simulink model "so3_ballpark"  (R2024b)
settings: Solver=FixedStepAuto  StartTime=0.0  StopTime=80  FixedStep=0.0001  RelTol=1e-3
values from neighbouring files (symbols this model uses):
  cube_length = 0.3    [s03_ballpark_init.m]
  cube_mass = 3    [s03_ballpark_init.m]
  Kr = 0.3    [s03_ballpark_init.m]
  Kw = 0.5*Kr    (= 0.15)    [s03_ballpark_init.m]
  q_des = eul2quat(desiered_rot_euler)    [s03_ballpark_init.m]
  T = 0.05    [s03_ballpark_init.m]    (also in thruster_mapper.m = 0.1)
  thruster_matrix = [ ... (first row only)    [s03_ballpark_init.m]    (also in thruster_mapper.m)
  X_0 = [ ... (first row only)    [s03_ballpark_init.m]
undefined symbols (not defined in the file or in its folder): X, Y, Z
libraries: simulink x24, nesl_utility x18, sm_lib x5
settings Model: Creator=user  LastModifiedBy=user
settings OptimizationCC: BlockReduction=off  DefaultParameterBehavior=Inlined  BufferReuse=off

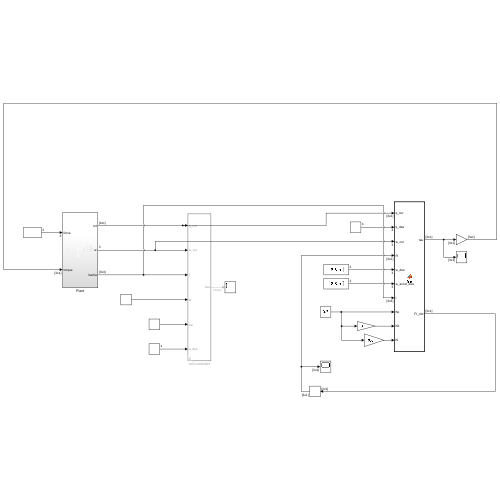
[thumbnail: Simulink's stored preview of the top-level diagram]
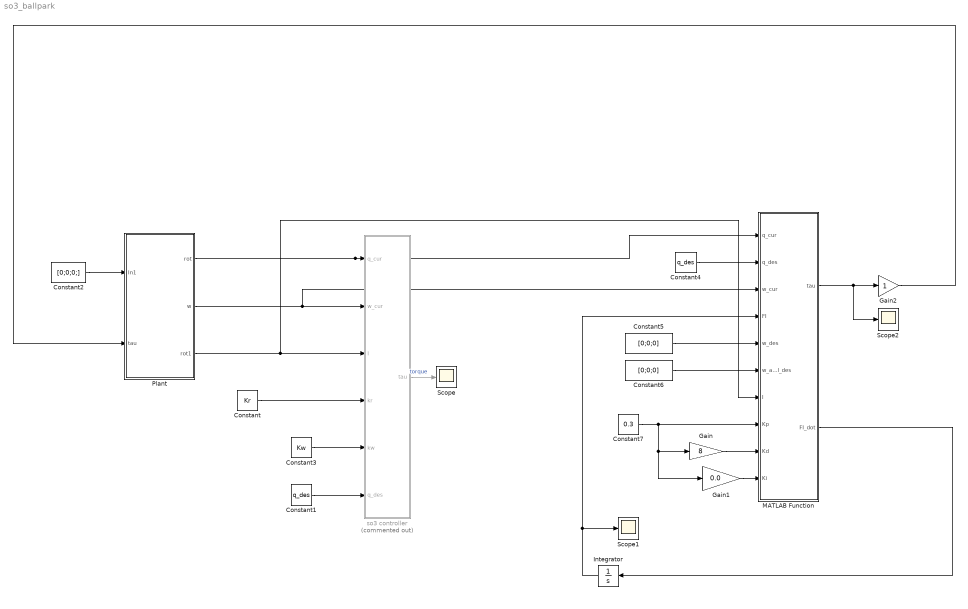
== system so3_ballpark ==
  Constant : Constant  Value=Kr
  Constant1 : Constant  Value=q_des
  Constant2 : Constant  Value=[0;0;0;]
  Constant3 : Constant  Value=Kw
  Constant4 : Constant  Value=q_des
  Constant5 : Constant  Value=[0;0;0]
  Constant6 : Constant  Value=[0;0;0]
  Constant7 : Constant  Value=0.3
  Gain : Gain  Gain=8
  Gain1 : Gain  Gain=0.0
  Gain2 : Gain
  Integrator : Integrator  InitialCondition=[0;0;0]
  MATLAB Function : MATLAB Function  TreatAsAtomicUnit=on  SystemSampleTime=T
  Plant : Subsystem
  Scope : Scope
  Scope1 : Scope
  Scope2 : Scope
  so3 controller : MATLAB Function  Commented=on  TreatAsAtomicUnit=on
  wires:
  so3 controller/1(tau) -> Scope/1  "torque"
  Plant/1(rot) -> MATLAB Function/1(q_cur), so3 controller/1(q_cur)
  Plant/2(w) -> MATLAB Function/3(w_cur), so3 controller/2(w_cur)
  Constant/1 -> so3 controller/4(kr)
  Constant1/1 -> so3 controller/6(q_des)
  Plant/3(rot1) -> MATLAB Function/7(I), so3 controller/3(I)
  Constant2/1 -> Plant/1(In1)
  Constant3/1 -> so3 controller/5(kw)
  MATLAB Function/2(FI_dot) -> Integrator/1
  Integrator/1 -> Scope1/1, MATLAB Function/4(FI)
  Constant4/1 -> MATLAB Function/2(q_des)
  Constant5/1 -> MATLAB Function/5(w_des)
  Constant6/1 -> MATLAB Function/6(w_accel_des)
  Constant7/1 -> Gain1/1, Gain/1, MATLAB Function/8(Kp)
  Gain/1 -> MATLAB Function/9(Kd)
  Gain1/1 -> MATLAB Function/10(Ki)
  MATLAB Function/1(tau) -> Scope2/1, Gain2/1
  Gain2/1 -> Plant/2(tau)

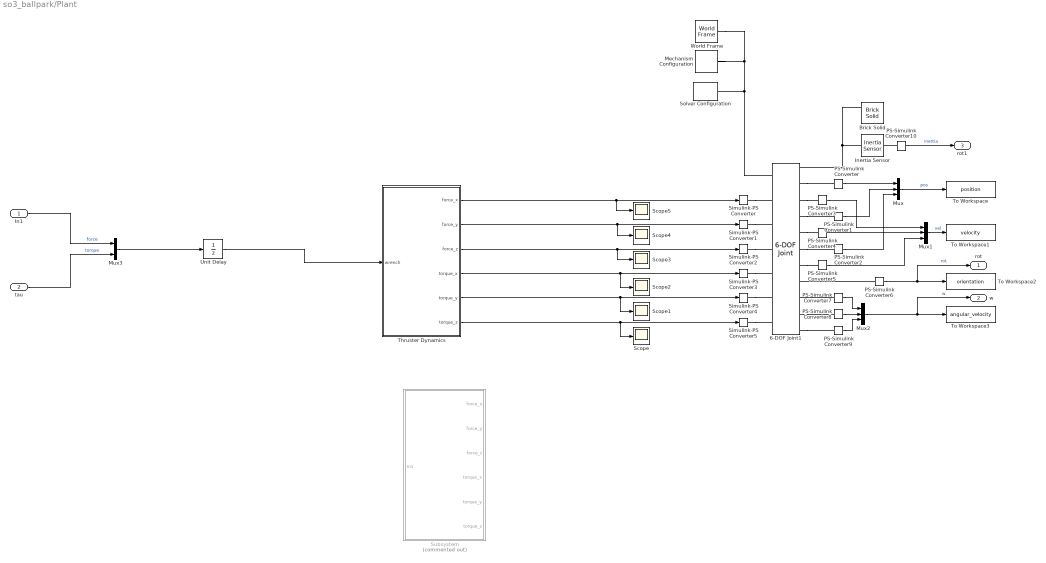
== system so3_ballpark/Plant ==
  In1 : Inport
  tau : Inport  Port=2
  6-DOF Joint1 : sm_lib/Joints/6-DOF Joint  JointMode=Normal  CompositeWrenchDir=FollowerOnBase  CompositeWrenchFrame=BaseFrame  SenseConstraintForce=off  SenseConstraintTorque=off  SenseTotalForce=off  SenseTotalTorque=off  PxPositionTargetSpecify=on  PxPositionTargetPriority=High  PxPositionTargetValue=X_0(1)  PxPositionTargetValueUnits=m  PxVelocityTargetSpecify=on  PxVelocityTargetPriority=High  PxVelocityTargetValue=X_0(4)  PxVelocityTargetValueUnits=m/s  PxEquilibriumPosition=0  PxEquilibriumPositionUnits=m  PxSpringStiffness=0  PxSpringStiffnessUnits=N/m  PxDampingCoefficient=0  PxDampingCoefficientUnits=N/(m/s)  PxLowerLimitSpecify=off  PxLowerLimitBound=-1  PxLowerLimitBoundUnits=m  PxLowerLimitStiffness=1e6  PxLowerLimitStiffnessUnits=N/m  PxLowerLimitDamping=1e3  PxLowerLimitDampingUnits=N/(m/s)  PxLowerLimitTransitionRegionWidth=1e-4  PxLowerLimitTransitionRegionWidthUnits=m  PxUpperLimitSpecify=off  PxUpperLimitBound=1  PxUpperLimitBoundUnits=m  PxUpperLimitStiffness=1e6  PxUpperLimitStiffnessUnits=N/m  PxUpperLimitDamping=1e3  PxUpperLimitDampingUnits=N/(m/s)  PxUpperLimitTransitionRegionWidth=1e-4  PxUpperLimitTransitionRegionWidthUnits=m  PxTorqueActuationMode=InputTorque  PxMotionActuationMode=ComputedMotion  PxSensePosition=on  PxSenseVelocity=on  PxSenseAcceleration=off  PxSenseTorqueForce=off  PxSenseLowerLimitTorqueForce=off  PxSenseUpperLimitTorqueForce=off  PyPositionTargetSpecify=on  PyPositionTargetPriority=High  PyPositionTargetValue=X_0(2)  PyPositionTargetValueUnits=m  PyVelocityTargetSpecify=on  PyVelocityTargetPriority=High  PyVelocityTargetValue=X_0(5)  PyVelocityTargetValueUnits=m/s  PyEquilibriumPosition=0  PyEquilibriumPositionUnits=m  PySpringStiffness=0  PySpringStiffnessUnits=N/m  PyDampingCoefficient=0  PyDampingCoefficientUnits=N/(m/s)  PyLowerLimitSpecify=off  PyLowerLimitBound=-1  PyLowerLimitBoundUnits=m  PyLowerLimitStiffness=1e6  PyLowerLimitStiffnessUnits=N/m  PyLowerLimitDamping=1e3  PyLowerLimitDampingUnits=N/(m/s)  PyLowerLimitTransitionRegionWidth=1e-4  PyLowerLimitTransitionRegionWidthUnits=m  PyUpperLimitSpecify=off  PyUpperLimitBound=1  PyUpperLimitBoundUnits=m  PyUpperLimitStiffness=1e6  PyUpperLimitStiffnessUnits=N/m  PyUpperLimitDamping=1e3  PyUpperLimitDampingUnits=N/(m/s)  PyUpperLimitTransitionRegionWidth=1e-4  PyUpperLimitTransitionRegionWidthUnits=m  PyTorqueActuationMode=InputTorque  PyMotionActuationMode=ComputedMotion  PySensePosition=on  PySenseVelocity=on  PySenseAcceleration=off  PySenseTorqueForce=off  PySenseLowerLimitTorqueForce=off  PySenseUpperLimitTorqueForce=off  PzPositionTargetSpecify=on  PzPositionTargetPriority=High  PzPositionTargetValue=X_0(3)  PzPositionTargetValueUnits=m  PzVelocityTargetSpecify=on  PzVelocityTargetPriority=High  PzVelocityTargetValue=X_0(6)  PzVelocityTargetValueUnits=m/s  PzEquilibriumPosition=0  PzEquilibriumPositionUnits=m  PzSpringStiffness=0  PzSpringStiffnessUnits=N/m  PzDampingCoefficient=0  PzDampingCoefficientUnits=N/(m/s)  PzLowerLimitSpecify=off  PzLowerLimitBound=-1  PzLowerLimitBoundUnits=m  PzLowerLimitStiffness=1e6  PzLowerLimitStiffnessUnits=N/m  PzLowerLimitDamping=1e3  PzLowerLimitDampingUnits=N/(m/s)  PzLowerLimitTransitionRegionWidth=1e-4  PzLowerLimitTransitionRegionWidthUnits=m  PzUpperLimitSpecify=off  PzUpperLimitBound=1  PzUpperLimitBoundUnits=m  PzUpperLimitStiffness=1e6  PzUpperLimitStiffnessUnits=N/m  PzUpperLimitDamping=1e3  PzUpperLimitDampingUnits=N/(m/s)  PzUpperLimitTransitionRegionWidth=1e-4  PzUpperLimitTransitionRegionWidthUnits=m  PzTorqueActuationMode=InputTorque  PzMotionActuationMode=ComputedMotion  PzSensePosition=on  PzSenseVelocity=on  PzSenseAcceleration=off  PzSenseTorqueForce=off  PzSenseLowerLimitTorqueForce=off  PzSenseUpperLimitTorqueForce=off  SphPositionTargetSpecify=on  SphPositionTargetPriority=High  SphPositionTargetRotationMethod=RotationSequence  SphPositionTargetFollAlignAxisA=+X  SphPositionTargetBaseAlignAxisA=+Y  SphPositionTargetFollAlignAxisB=+Y  SphPositionTargetBaseAlignAxisB=+Z  SphPositionTargetRotationStandardAxis=+Z  SphPositionTargetRotationAngle=0  SphPositionTargetRotationAngleUnits=deg  SphPositionTargetRotationArbitraryAxis=[0 0 1]  SphPositionTargetRotationSequenceAxes=FollowerAxes  SphPositionTargetRotationSequence=XYZ  SphPositionTargetRotationSequenceAngles=X_0(7:9)'  SphPositionTargetRotationSequenceAnglesUnits=deg  SphPositionTargetRotationMatrix=[1 0 0;0 1 0;0 0 1]  SphPositionTargetQuaternion=[1 0 0 0]  SphVelocityTargetSpecify=on  SphVelocityTargetPriority=High  SphVelocityTargetValue=X_0(10:12)'  SphVelocityTargetValueUnits=deg/s  SphVelocityTargetInFollowerFrame=on  SphEqPosRotationMethod=None  SphEqPosFollAlignAxisA=+X  SphEqPosBaseAlignAxisA=+Y  SphEqPosFollAlignAxisB=+Y  SphEqPosBaseAlignAxisB=+Z  SphEqPosRotationStandardAxis=+Z  SphEqPosRotationAngle=0  SphEqPosRotationAngleUnits=deg  SphEqPosRotationArbitraryAxis=[0 0 1]  SphEqPosRotationSequenceAxes=FollowerAxes  SphEqPosRotationSequence=XYX  SphEqPosRotationSequenceAngles=[0 0 0]  SphEqPosRotationSequenceAnglesUnits=deg  SphEqPosRotationMatrix=[1 0 0;0 1 0;0 0 1]  SphEqPosQuaternion=[1 0 0 0]  SphSpringStiffness=0  SphSpringStiffnessUnits=N*m/deg  SphDampingCoefficient=0  SphDampingCoefficientUnits=N*m/(deg/s)  SphLowerLimitSpecify=off  SphLowerLimitBound=15  SphLowerLimitBoundUnits=deg  SphLowerLimitStiffness=1e4  SphLowerLimitStiffnessUnits=N*m/deg  SphLowerLimitDamping=10  SphLowerLimitDampingUnits=N*m/(deg/s)  SphLowerLimitTransitionRegionWidth=0.1  SphLowerLimitTransitionRegionWidthUnits=deg  SphUpperLimitSpecify=off  SphUpperLimitBound=45  SphUpperLimitBoundUnits=deg  SphUpperLimitStiffness=1e4  SphUpperLimitStiffnessUnits=N*m/deg  SphUpperLimitDamping=10  SphUpperLimitDampingUnits=N*m/(deg/s)  SphUpperLimitTransitionRegionWidth=0.1  SphUpperLimitTransitionRegionWidthUnits=deg  SphTorqueActuationMode=InputTorque  SphActuateTorqueX=on  SphActuateTorqueY=on  SphActuateTorqueZ=on  SphActuateTorque=off  SphActuationFrame=BaseFrame  SphSensePosition=on  SphSenseVelocityX=on  SphSenseVelocityY=on  SphSenseVelocityZ=on  SphSenseVelocity=off  SphSenseAccelerationX=off  SphSenseAccelerationY=off  SphSenseAccelerationZ=off  SphSenseAcceleration=off  SphSenseLowerLimitTorqueMag=off  SphSenseUpperLimitTorqueMag=off  SphSensingFrame=BaseFrame
  Brick Solid : sm_lib/Body Elements/Brick Solid  BrickDimensions=[cube_length cube_length cube_length]  BrickDimensionsUnits=m  ExportEntireGeometry=on  InertiaType=CalculateFromGeometry  BasedOnType=Mass  Density=1000  DensityUnits=kg/m^3  Mass=cube_mass  MassUnits=kg  CenterOfMass=[0 0 0]  CenterOfMassUnits=m  MomentsOfInertia=[1 1 1]  MomentsOfInertiaUnits=kg*m^2  ProductsOfInertia=[0 0 0]  ProductsOfInertiaUnits=kg*m^2  GraphicType=FromGeometry  MarkerShape=Sphere  MarkerSize=10  GraphicVisPropType=SimpleVisualProperties  GraphicDiffuseColor=[0.5 0.5 0.5]  GraphicOpacity=1  GraphicSpecularColor=[0.5 0.5 0.5 1.0]  GraphicAmbientColor=[0.15 0.15 0.15 1.0]  GraphicEmissiveColor=[0.0 0.0 0.0 1.0]  GraphicShininess=75  DoExposeReferenceFrame=on  SerializedFrames=<Frames><Frame><Id>Frame1</Id><Value><Name>F1</Name><Origin><Source>ReferenceFrame</Source><FeatureName></FeatureName></Origin><PrimaryAxis><DefinedDirection>+Z</DefinedDirection><Source>ReferenceFrame</Source><SourceDirection>+Z</SourceDirection><FeatureName></FeatureName></PrimaryAxis><SecondaryAxis><DefinedDirection>+X</DefinedDirection><Source>ReferenceFrame</Source><SourceDirection>+X</SourceDirection><FeatureName></FeatureName></SecondaryAxis></Value></Frame></Frames>
  Inertia Sensor : sm_lib/Body Elements/Inertia Sensor  SensorExtent=BodyGroup  SpanWeldJoints=off  ExcludeGroundedBodies=off  MeasurementFrame=Attached  SenseMass=off  SenseCenterOfMass=off  SenseInertiaMatrix=on  SenseCenteredInertiaMatrix=off  SensePrincipalInertiaMatrix=off  SenseRotationMatrix=off  GraphicType=PrincipalInertiaFrame  PrincipalInertiaFrameSize=20  GraphicVisPropType=SimpleVisualProperties  GraphicDiffuseColor=[0.5 0.5 0.5]  GraphicOpacity=1  GraphicSpecularColor=[0.5 0.5 0.5 1.0]  GraphicAmbientColor=[0.15 0.15 0.15 1.0]  GraphicEmissiveColor=[0.0 0.0 0.0 1.0]  GraphicShininess=75
  Mechanism Configuration : sm_lib/Utilities/Mechanism Configuration  UniformGravity=Constant  GravityVector=[0 0 0]  GravityVectorUnits=m/s^2  LinearizationDelta=0.001  JointModeTransitionNonlinearIterations=2
  Mux : Mux  Inputs=3
  Mux1 : Mux  Inputs=3
  Mux2 : Mux  Inputs=3
  Mux3 : Mux  Inputs=2
  PS-Simulink Converter{,1..10} (11 alike) : nesl_utility/PS-Simulink Converter  PhysicalDomain=network_engine_domain  SubClassName=ps_output  LeftPortType=input  RightPortType=output  PseudoPeriodic=off  Frequencies=[]  VectorFormat=inherit  Unit=inherit  AffineConversion=off
  Scope{,1..5} (6 alike) : Scope
  Simulink-PS Converter{,1..5} (6 alike) : nesl_utility/Simulink-PS Converter  PhysicalDomain=network_engine_domain  SubClassName=ps_input  LeftPortType=input  RightPortType=output  PseudoPeriodic=off  Frequencies=[]  NoiseDistribution=none  NoiseParameters=[]  Unit=1  AffineConversion=off  FilteringAndDerivatives=provide  SimscapeFilterOrder=1  InputFilterTimeConstant=0.001  UdotUserProvided=0
  Solver Configuration : nesl_utility/Solver Configuration  PhysicalDomain=network_engine_domain  SubClassName=solver  LeftPortType=input  RightPortType=generic  Tones=[]  Harmonics=[]  SimulateNoise=off  Profile=off  UseLocalSampling=off  EnableSwitchedLinearOptims=on  FrequencyDomain=off  UseCCode=off  RelTol=0.001  AbsTol=0.001  MinStep=1e-09  ToWorkspace=off  RevertToSquareIcSolve=off  NumHomotopyIterations=100  PhasorMode=off  PhasorModeNumHarmonics=1  ConsistencySolver=NEWTON_XTOL_AFTER_FTOL  IndexReductionMethod=DerivativeReplacement  DoDC=off  ResidualTolerance=1e-09  ConsistencyTolSource=GLOBAL  ConsistencyAbsTol=0.001  ConsistencyRelTol=0.001  ConsistencyTolFactor=0.001  UseLocalSolver=off  LocalSolverChoice=NE_BACKWARD_EULER_ADVANCER  ResolveIndetEquations=on  FunctionEvalNumThread=1  LocalSolverSampleTime=0.001  DoFixedCost=off  MaxNonlinIter=3  MaxModeIter=2  ComputeImpulses=off  ImpulseIterations=2  LinearAlgebra=auto  LinearAlgebraNumThread=0  EquationFormulation=NE_TIME_EF  DelaysMemoryBudget=1024  AutomaticFiltering=on  FilteringTimeConstant=0.001  PartitionStorageMethod=AS_NEEDED  PartitionMemoryBudget=1024  PartitionMethod=ROBUST  MultibodyUseLocalSolver=off  MultibodyLocalSolverChoice=ODE1  MultibodyLocalSolverSampleTime=0.001
  Subsystem : Subsystem  Commented=on
  Thruster Dynamics : Subsystem
  To Workspace : ToWorkspace  VariableName=position  SampleTime=-1
  To Workspace1 : ToWorkspace  VariableName=velocity  SampleTime=-1
  To Workspace2 : ToWorkspace  VariableName=orientation  SampleTime=-1
  To Workspace3 : ToWorkspace  VariableName=angular_velocity  SampleTime=-1
  Unit Delay : UnitDelay  SampleTime=-1  HasFrameUpgradeWarning=on
  World Frame : sm_lib/Frames and Transforms/World Frame
  rot : Outport
  w : Outport  Port=2
  rot1 : Outport  Port=3
  wires:
  PS-Simulink Converter4/1 -> Mux1/2
  Mux1/1 -> To Workspace1/1  "vel"
  PS-Simulink Converter5/1 -> Mux1/3
  PS-Simulink Converter8/1 -> Mux2/2
  Mux/1 -> To Workspace/1  "pos"
  PS-Simulink Converter9/1 -> Mux2/3
  PS-Simulink Converter/1 -> Mux/1
  PS-Simulink Converter7/1 -> Mux2/1
  PS-Simulink Converter6/1 -> rot/1, To Workspace2/1  "rot"
  PS-Simulink Converter1/1 -> Mux/2
  PS-Simulink Converter3/1 -> Mux1/1
  Mux2/1 -> w/1, To Workspace3/1  "w"
  PS-Simulink Converter2/1 -> Mux/3
  In1/1 -> Mux3/1  "force"
  tau/1 -> Mux3/2  "torque"
  PS-Simulink Converter10/1 -> rot1/1  "inertia"
  Mux3/1 -> Unit Delay/1
  Thruster Dynamics/6(torque_z) -> Scope/1, Simulink-PS Converter5/1
  Thruster Dynamics/1(force_x) -> Scope5/1, Simulink-PS Converter/1
  Thruster Dynamics/4(torque_x) -> Scope2/1, Simulink-PS Converter3/1
  Thruster Dynamics/3(force_z) -> Scope3/1, Simulink-PS Converter2/1
  Thruster Dynamics/5(torque_y) -> Scope1/1, Simulink-PS Converter4/1
  Thruster Dynamics/2(force_y) -> Scope4/1, Simulink-PS Converter1/1
  Unit Delay/1 -> Thruster Dynamics/1(wrench)
  connections:
  Simulink-PS Converter2/RConn1 -- 6-DOF Joint1/LConn4
  Simulink-PS Converter/RConn1 -- 6-DOF Joint1/LConn2
  6-DOF Joint1/RConn7 -- PS-Simulink Converter5/LConn1
  Simulink-PS Converter1/RConn1 -- 6-DOF Joint1/LConn3
  6-DOF Joint1/RConn5 -- PS-Simulink Converter4/LConn1
  6-DOF Joint1/RConn11 -- PS-Simulink Converter9/LConn1
  6-DOF Joint1/RConn6 -- PS-Simulink Converter2/LConn1
  Brick Solid/LConn1 -- Inertia Sensor/LConn1 -- 6-DOF Joint1/RConn1
  6-DOF Joint1/RConn9 -- PS-Simulink Converter7/LConn1
  World Frame/RConn1 -- 6-DOF Joint1/LConn1 -- Solver Configuration/RConn1 -- Mechanism Configuration/RConn1
  6-DOF Joint1/RConn10 -- PS-Simulink Converter8/LConn1
  Simulink-PS Converter3/RConn1 -- 6-DOF Joint1/LConn5
  Simulink-PS Converter4/RConn1 -- 6-DOF Joint1/LConn6
  6-DOF Joint1/RConn4 -- PS-Simulink Converter1/LConn1
  6-DOF Joint1/RConn3 -- PS-Simulink Converter3/LConn1
  6-DOF Joint1/RConn2 -- PS-Simulink Converter/LConn1
  Simulink-PS Converter5/RConn1 -- 6-DOF Joint1/LConn7
  PS-Simulink Converter6/LConn1 -- 6-DOF Joint1/RConn8
  PS-Simulink Converter10/LConn1 -- Inertia Sensor/RConn1

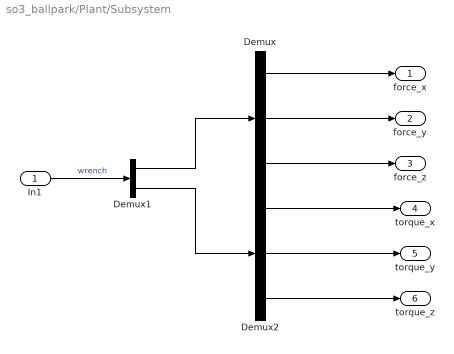
== system so3_ballpark/Plant/Subsystem ==
  In1 : Inport
  Demux : Demux  Outputs=3
  Demux1 : Demux  Outputs=2
  Demux2 : Demux  Outputs=3
  force_x : Outport
  force_y : Outport  Port=2
  force_z : Outport  Port=3
  torque_x : Outport  Port=4
  torque_y : Outport  Port=5
  torque_z : Outport  Port=6
  wires:
  Demux2/3 -> torque_z/1
  Demux/1 -> force_x/1
  Demux/3 -> force_z/1
  Demux/2 -> force_y/1
  Demux2/2 -> torque_y/1
  Demux2/1 -> torque_x/1
  In1/1 -> Demux1/1  "wrench"
  Demux1/1 -> Demux/1
  Demux1/2 -> Demux2/1

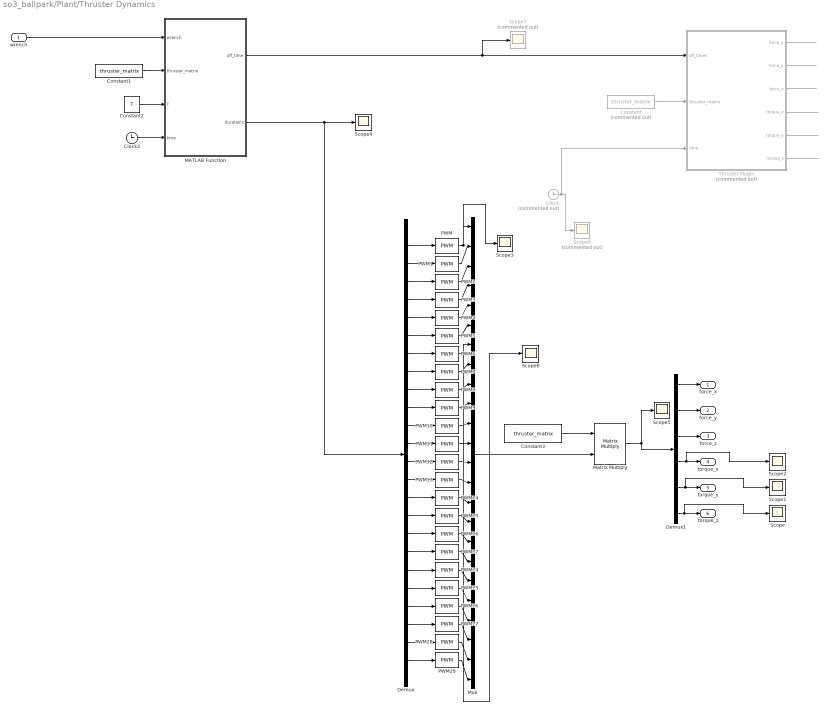
== system so3_ballpark/Plant/Thruster Dynamics ==
  wrench : Inport
  Clock : Clock  Commented=on
  Clock3 : Clock
  Constant : Constant  Commented=on  Value=thruster_matrix
  Constant1 : Constant  Value=thruster_matrix
  Constant2 : Constant  Value=T
  Constant3 : Constant  Value=thruster_matrix
  Demux : Demux  Outputs=24
  Demux1 : Demux  Outputs=6
  MATLAB Function : MATLAB Function  TreatAsAtomicUnit=on  SystemSampleTime=T
  Matrix Multiply : Product  Multiplication=Matrix(*)
  Mux : Mux  Inputs=24
  PWM{,1..17,24..29} (24 alike) : simulink/Discontinuities/PWM  DisableCoverage=on  Period=T  InitialDelay=0  DisallowZeroDutyCycle=off  RunAtFixedTimeIntervals=on  SampleTime=T/100
  Scope{,1..5,8} (7 alike) : Scope
  Scope6 : Scope  Commented=on
  Scope7 : Scope  Commented=on
  Thruster Plugin : MATLAB Function  Commented=on  TreatAsAtomicUnit=on
  force_x : Outport
  force_y : Outport  Port=2
  force_z : Outport  Port=3
  torque_x : Outport  Port=4
  torque_y : Outport  Port=5
  torque_z : Outport  Port=6
  wires:
  Thruster Plugin/6(torque_z) -> ?
  Thruster Plugin/4(torque_x) -> ?
  wrench/1 -> MATLAB Function/1(wrench)
  Constant/1 -> Thruster Plugin/2(thruster_matrix)
  Thruster Plugin/2(force_y) -> ?
  Constant2/1 -> MATLAB Function/3(T)
  Thruster Plugin/1(force_x) -> ?
  Thruster Plugin/5(torque_y) -> ?
  Clock/1 -> Scope6/1, Thruster Plugin/3(time)
  Constant1/1 -> MATLAB Function/2(thruster_matrix)
  Clock3/1 -> MATLAB Function/4(time)
  Thruster Plugin/3(force_z) -> ?
  Demux/1 -> PWM/1
  MATLAB Function/1(off_time) -> Scope7/1, Thruster Plugin/1(off_times)
  MATLAB Function/2(durations) -> Scope4/1, Demux/1
  Demux/2 -> PWM1/1
  Demux/4 -> PWM3/1
  Demux/3 -> PWM2/1
  Demux/8 -> PWM7/1
  Demux/6 -> PWM5/1
  Demux/7 -> PWM6/1
  Demux/5 -> PWM4/1
  Demux/12 -> PWM11/1
  Demux/14 -> PWM13/1
  Demux/15 -> PWM14/1
  Demux/11 -> PWM10/1
  Demux/13 -> PWM12/1
  Demux/10 -> PWM9/1
  Demux/16 -> PWM15/1
  Demux/9 -> PWM8/1
  Demux/24 -> PWM29/1
  Demux/21 -> PWM26/1
  Demux/23 -> PWM28/1
  Demux/18 -> PWM17/1
  Demux/22 -> PWM27/1
  Demux/20 -> PWM25/1
  Demux/19 -> PWM24/1
  Demux/17 -> PWM16/1
  PWM/1 -> Scope3/1, Mux/1
  PWM1/1 -> Mux/2
  PWM2/1 -> Mux/3
  PWM3/1 -> Mux/4
  PWM4/1 -> Mux/5
  PWM5/1 -> Mux/6
  PWM6/1 -> Scope8/1, Mux/7
  PWM7/1 -> Mux/8
  PWM8/1 -> Mux/9
  PWM9/1 -> Mux/10
  PWM10/1 -> Mux/11
  PWM11/1 -> Mux/12
  PWM12/1 -> Mux/13
  PWM13/1 -> Mux/14
  PWM14/1 -> Mux/15
  PWM15/1 -> Mux/16
  PWM16/1 -> Mux/17
  PWM17/1 -> Mux/18
  PWM24/1 -> Mux/19
  PWM25/1 -> Mux/20
  PWM26/1 -> Mux/21
  PWM27/1 -> Mux/22
  PWM28/1 -> Mux/23
  PWM29/1 -> Mux/24
  Mux/1 -> Matrix Multiply/2
  Constant3/1 -> Matrix Multiply/1
  Matrix Multiply/1 -> Scope5/1, Demux1/1
  Demux1/1 -> force_x/1
  Demux1/2 -> force_y/1
  Demux1/3 -> force_z/1
  Demux1/4 -> Scope2/1, torque_x/1
  Demux1/5 -> Scope1/1, torque_y/1
  Demux1/6 -> Scope/1, torque_z/1

== matlab function so3_ballpark/Plant/Thruster Dynamics/Thruster Plugin ==
  data: force_x output; force_y output; off_times input; thruster_matrix input; time input; force_z output; torque_x output; torque_y output; torque_z output
function [force_x, force_y, force_z, torque_x, torque_y, torque_z]= fcn(off_times, thruster_matrix, time)

n_thrusters = length(off_times);
firing_thrusters = zeros(n_thrusters, n_thrusters);

for i = 1:n_thrusters
    % disable thruster if it should not be fired
    if off_times(i) > (time+0.002)
        firing_thrusters(i, i) = 1;
    end
end

output = thruster_matrix * firing_thrusters;

force_x = sum(output(1,:));
force_y = sum(output(2,:));
force_z = sum(output(3,:));

torque_x = sum(output(4,:));
torque_y = sum(output(5,:));
torque_z = sum(output(6,:));

== matlab function so3_ballpark/so3 controller ==
  data: q_cur input; w_cur input; I input; kr input; kw input; q_des input; tau output
function tau = fcn(q_cur, w_cur, I, kr, kw, q_des)

w_des = [
    0;
    0;
    0
    ];

R_cur = quat2rotm(q_cur');
R_des = quat2rotm(q_des');

R_e = R_des' * R_cur;

theta = acos((trace(R_e) - 1)/2);
if abs(theta - pi) < 1e-3  % Near 180 degrees
    % Special handling for numerical stability
    q_err = quatmult(quatinv(q_des), q_cur);  % error quaternion
    if q_err(1) < 0  % shortest path
        q_err = -q_err;
    end
    e_vec = q_err(2:4);
else
    e_R = 0.5 .* (R_e - R_e');
    
    e_vec = [
        e_R(3,2);
        e_R(1,3);
        e_R(2,1)
        ];
end

e_w = w_cur - (R_cur' * (R_des * w_des));

tau = -kr .* e_vec - kw*e_w + cross(w_cur, I * w_cur)

== matlab function so3_ballpark/Plant/Thruster Dynamics/MATLAB Function ==
  data: wrench input; off_time output; thruster_matrix input; T input; time input; durations output
function [off_time, durations]= fcn(wrench, thruster_matrix, T, time)

n_thrusters = length(thruster_matrix');

opts = optimoptions('lsqlin', 'Algorithm', 'active-set');

t = lsqlin( ...
    eye(24), ...               % H: Identity matrix for norm minimization
    zeros(24,1), ...           % f: zero linear term
    [], [], ...                % No inequality constraints
    thruster_matrix, wrench .* T, ... % Aeq * x = beq
    zeros(24,1), ones(24,1)*T*0.7, ...       % lb: x >= 0, ub: no upper bound
    zeros(24,1), opts);    

for i = 1:length(t)
    if t(i) > 0.7*T
        t(i) = 0.7*T;
    end

    if t(i) < 0.1*T
        t(i) = 0;
    end


end

off_time = time * ones(24,1) +  t;
durations = t;

== matlab function so3_ballpark/MATLAB Function ==
  data: tau output; q_cur input; q_des input; w_cur input; FI input; w_des input; w_accel_des input; I input; FI_dot output; Kp input; Kd input; Ki input
function [tau, FI_dot]= fcn(q_cur, q_des, w_cur, FI, w_des, w_accel_des, I, Kp, Kd, Ki)

R_cur = quat2rotm(q_cur');
R_des = quat2rotm(q_des');

Q = R_des' * R_cur;

K = eye(3);

e = eye(3);

SK = zeros(3,1);

for i = 1:3
    SK = SK + K(i,i)* cross(Q'*e(:,i), e(:,i));
end

w = (w_cur - Q'*w_des);

W = [
    0,      -w(3),      w(2);
    w(3),       0,     -w(1);
    -w(2),   w(1),         0;
    ];

FI_dot = I \ (Kp*SK + Kd*w + cross(I*w_cur, FI));

tau = -Kp*SK -Ki*FI -Kd*w + I * (Q'*w_accel_des - w'*Q'*w_des) - cross(I*w_cur,Q'*w_des);
